simulink model "Sistema_Seguimiento_Con_Planta_Tipo_0"  (R2016a)
settings: Solver=VariableStepAuto  StartTime=0.0  StopTime=2  RelTol=1e-3
values from neighbouring files (symbols this model uses):
  Init_cond = [0 0 0]    [Final_2018.m]
undefined symbols (not defined in the file or in its folder): A, B, C, D
settings Model: Creator=adrie  LastModifiedBy=adrie
settings GRTTargetCC: GeneratePreprocessorConditionals=Use local settings

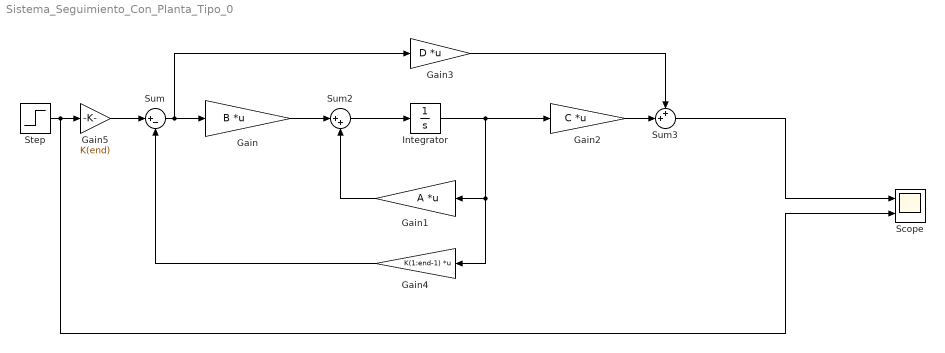
== system Sistema_Seguimiento_Con_Planta_Tipo_0 ==
  Gain : Gain  Gain=B  Multiplication=Matrix(K*u) (u vector)
  Gain1 : Gain  Gain=A  Multiplication=Matrix(K*u) (u vector)
  Gain2 : Gain  Gain=C  Multiplication=Matrix(K*u) (u vector)
  Gain3 : Gain  Gain=D  Multiplication=Matrix(K*u) (u vector)
  Gain4 : Gain  Gain=K(1:end-1)  Multiplication=Matrix(K*u) (u vector)
  Gain5 : Gain  Gain=K(end)
  Integrator : Integrator  InitialCondition=Init_cond
  Scope : Scope  NumInputPorts=2
  Step : Step  Time=0  SampleTime=0
  Sum : Sum  Inputs=|+-
  Sum2 : Sum  Inputs=|++
  Sum3 : Sum  Inputs=++|
  wires:
  Gain/1 -> Sum2/1
  Sum2/1 -> Integrator/1
  Gain1/1 -> Sum2/2
  Integrator/1 -> Gain2/1, Gain4/1, Gain1/1
  Gain2/1 -> Sum3/2
  Gain3/1 -> Sum3/1
  Sum3/1 -> Scope/1
  Sum/1 -> Gain3/1, Gain/1
  Gain4/1 -> Sum/2
  Step/1 -> Scope/2, Gain5/1
  Gain5/1 -> Sum/1
